simulink model "doc_design_iteration_viterbi_visualize"  (R2014a)
settings: Solver=FixedStepDiscrete  SolverMode=SingleTasking  StartTime=0.0  StopTime=inf  RelTol=1e-3
PostLoadFcn:
  | if ~exist('EbNo'),EbNo=6;end
  | if ~exist('MaxNumBits'),MaxNumBits=1e7;end;
  | if ~exist('MaxNumErrs'),MaxNumErrs=1e3;end;
  | if ~exist('Seed'),Seed=211;end;
  | 
  | Param.BitsPerFrame=186;
  | Param.Len1=186+6;
  | pre1=0.5*((-1).^(0:1:99)+1);
  | pre2=0.5*((-1).^(1:100)+1);
  | Param.Preamble=complex([pre1 0.0 pre2].');
  | 
  | clear pre1 pre2
values from neighbouring files (symbols this model uses):
  EbNo = getTestParameter(obj,'EbNo')    [GrayCodedMod_EbNo_M.m]    (also in GrayCodedModulation2.m; commdoc_code.m = 10; commdoc_gray.m = 10; commdoc_mcurves.m = EbNoVec(idxEbNo))
libraries: commdigbbndpm3 x2, commcnvcod2 x2, commchan3 x1, commsink2 x1, commrandsrc2 x1, dspstat3 x1, dspmathops x1
settings Model: Creator=The MathWorks Inc.
settings OptimizationCC: ExpressionDepthLimit=2147483647
settings DebuggingCC: UnderspecifiedInitializationDetection=Classic  SolverPrmCheckMsg=none  StateNameClashWarn=warning

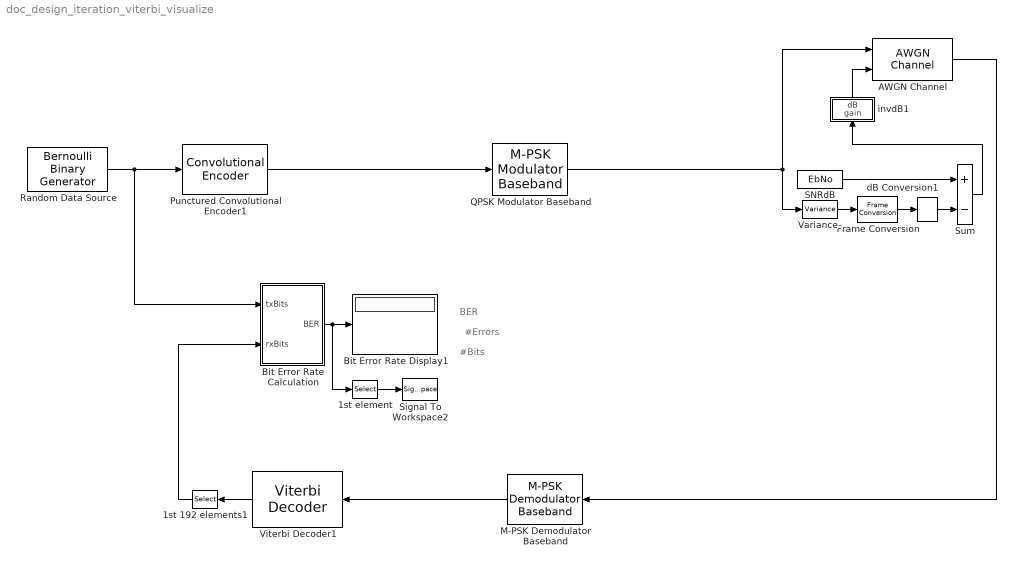
== system doc_design_iteration_viterbi_visualize ==
  note: BER
  note: #Bits
  note: #Errors
  1st 192 elements1 : Selector  NumberOfDimensions=2  InputPortWidth=3  IndexOptions=Index vector (dialog),Index vector (dialog)  Indices=1:186,1  OutputSizes=1,1
  1st element : Selector  InputPortWidth=3
  AWGN Channel : commchan3/AWGN Channel  InputProcessing=Columns as channels (frame based)  seed=67  noiseMode=Variance from port  EbNodB=10  EsNodB=15  SNRdB=10  bitsPerSym=1  Ps=1  Tsym=1e-6  variance=1
  Bit Error Rate Calculation : Subsystem
      mask Display: disp('Bit Error Rate\nCalculation');
  Bit Error Rate Display1 : Display
  Frame Conversion : FrameConversion  OutFrame=Sample-based
  M-PSK Demodulator Baseband : commdigbbndpm3/M-PSK Demodulator Baseband  M=4  Ph=pi/4  Dec=Gray  Mapping=[0 2 3 1]  OutType=Bit  DecType=Hard decision  VarSource=Dialog  Variance=1  outDtype1=boolean  outDtype2=Inherit via internal rule  derotateFactorWordLen=16
  Punctured Convolutional Encoder1 : commcnvcod2/Convolutional Encoder  trellis=poly2trellis(7, [171 133])  opMode=Terminate trellis by appending bits  DelayedResetAction=off  hasIniStPort=off  hasFinStPort=off  usePuncVector=on  punctureVector=reshape([1 0;1 1],4,1)  reset=Unused parameter value
  QPSK Modulator Baseband : commdigbbndpm3/M-PSK Modulator Baseband  M=4  InType=Bit  Enc=Gray  Mapping=[0 2 3 1]  Ph=pi/4  outDtype=double  outWordLen=16  outUDDataType=sfix(16)  outFracLenMode=Best precision  outFracLen=15
  Random Data Source : commrandsrc2/Bernoulli Binary Generator  P=0.5  seed=61  Ts=25/3e6  frameBased=on  sampPerFrame=186  orient=off  outDataType=boolean
  SNRdB : Constant  Value=EbNo
  Signal To Workspace2 : SignalToWorkspace  VariableName=ber
      settings: CopyFcn=dspblkcopystw(gcbh);  MaxDataPoints=3
  Sum : Sum  Inputs=+-  SaturateOnIntegerOverflow=on
  Variance : dspstat3/Variance  run=off  reset_popup=None  InputProcessing=Columns as channels (frame based)  directionMode=Each column  dimension=1  treatSBRowAsCol=on  roiEnable=off  roiType=Rectangles  roiPortion=Entire ROI  roiOutput=Individual statistics for each ROI  roiFlag=off  roundingMode=Floor  overflowMode=off
  Viterbi Decoder1 : commcnvcod2/Viterbi Decoder  trellis=poly2trellis(7, [171 133])  isPunctured=off  punctureVector=reshape([1 0;1 1],4,1)  erasures=off  dectype=Hard decision  runSigValErrCheck=off  nsdecb=4  smWordLength=16  tbdepth=34  opmode=Terminated  reset=off  outDataType=boolean  delayedResetAction=off
  dB Conversion1 : dspmathops/dB Conversion  dBtype=dB  intype=Power  R=1  fuzz=on
  invdB1 : Subsystem
      mask Display: disp('1/invdB')
  wires:
  Random Data Source/1 -> Bit Error Rate Calculation/1(txBits), Punctured Convolutional Encoder1/1
  Punctured Convolutional Encoder1/1 -> QPSK Modulator Baseband/1
  dB Conversion1/1 -> Sum/2
  Variance/1 -> Frame Conversion/1
  Frame Conversion/1 -> dB Conversion1/1
  invdB1/1(dB) -> AWGN Channel/2
  Sum/1 -> invdB1/1(gain)
  SNRdB/1 -> Sum/1
  QPSK Modulator Baseband/1 -> AWGN Channel/1, Variance/1
  M-PSK Demodulator Baseband/1 -> Viterbi Decoder1/1
  Bit Error Rate Calculation/1(BER) -> Bit Error Rate Display1/1, 1st element/1
  1st element/1 -> Signal To Workspace2/1
  Viterbi Decoder1/1 -> 1st 192 elements1/1
  1st 192 elements1/1 -> Bit Error Rate Calculation/2(rxBits)
  AWGN Channel/1 -> M-PSK Demodulator Baseband/1

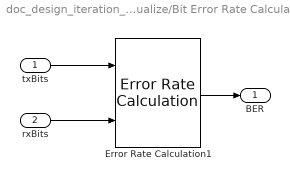
== system doc_design_iteration_viterbi_visualize/Bit Error Rate Calculation ==
  txBits : Inport
  rxBits : Inport  Port=2
  Error Rate Calculation1 : commsink2/Error Rate Calculation  N=0  st_delay=0  cp_mode=Entire frame  subframe=1:184  PMode=Port  WsName=ErrorVec  RsMode2=off  stop=on  numErr=MaxNumErrs  maxBits=MaxNumBits
  BER : Outport
  wires:
  txBits/1 -> Error Rate Calculation1/1
  Error Rate Calculation1/1 -> BER/1
  rxBits/1 -> Error Rate Calculation1/2

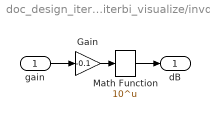
== system doc_design_iteration_viterbi_visualize/invdB1 ==
  gain : Inport
  Gain : Gain  Gain=-0.1  SaturateOnIntegerOverflow=on  OutDataTypeStr=Inherit: Same as input  ParamDataTypeStr=Inherit: Same as input
  Math Function : Math  Operator=10^u  SaturateOnIntegerOverflow=on
  dB : Outport
  wires:
  Gain/1 -> Math Function/1
  gain/1 -> Gain/1
  Math Function/1 -> dB/1
